simulink model "UIO_example_EEG"  (R2019b)
settings: Solver=FixedStepAuto  StartTime=0.0  StopTime=3  FixedStep=dt  RelTol=1e-3
values from neighbouring files (symbols this model uses):
  B2 = [68245 0 0;0 -2 0;0 0 2;0 232.75 0; 0 0 -232.75]    [UIO_adaptive_example.m]    (also in UIO_adaptive_example_2.m = [1;0;1;0]; UIO_adaptive_example_EEG.m = ones(opt_order,1); UIO_adaptive_example_EEG_Balas_2ch.m = ones(opt_order,1); UIO_adaptive_example_EEG_ch2.m = ones(opt_order,1))
  F = B2'*P/(C)    [UIO_adaptive_example_2.m]    (also in UIO_adaptive_example_EEG.m = B2'*P/(C_data{opt_order}); UIO_adaptive_example_EEG_ch2.m = B2'*P/(C_data{opt_order}); UIO_adaptive_example_EEG_ch2_DEAP.m = B2'*P/(C_data{opt_order}); UIO_adaptive_example_EEG_ch2_ECEO.m = B2'*P/(C_data{opt_order}))
  Gamma = 20    [UIO_adaptive_example_2.m]    (also in UIO_adaptive_example_EEG.m = 0.001; UIO_adaptive_example_EEG_ch2.m = loop(i); UIO_adaptive_example_EEG_ch2_DEAP.m = loop(i); UIO_adaptive_example_EEG_ch2_ECEO.m = loop(i))
  L = inv(P)*Y    [UIO_adaptive_example.m]    (also in UIO_adaptive_example_2.m; UIO_adaptive_example_EEG.m; UIO_adaptive_example_EEG_ch2.m; UIO_adaptive_example_EEG_ch2_DEAP.m)
  opt_order = 20    [UIO_adaptive_example_EEG.m]    (also in UIO_adaptive_example_EEG_Balas_2ch.m = 4; UIO_adaptive_example_EEG_ch2.m = 4; UIO_adaptive_example_EEG_ch2_DEAP.m = 4; UIO_adaptive_example_EEG_ch2_ECEO.m = 4)
settings Model: Creator=Tris  LastModifiedBy=Tris
settings DataIOCC: ExternalInput=Y_sim1, Y_sim2, Y_sim3, Y_sim4, Y_sim5, Y_sim6  LoadExternalInput=on

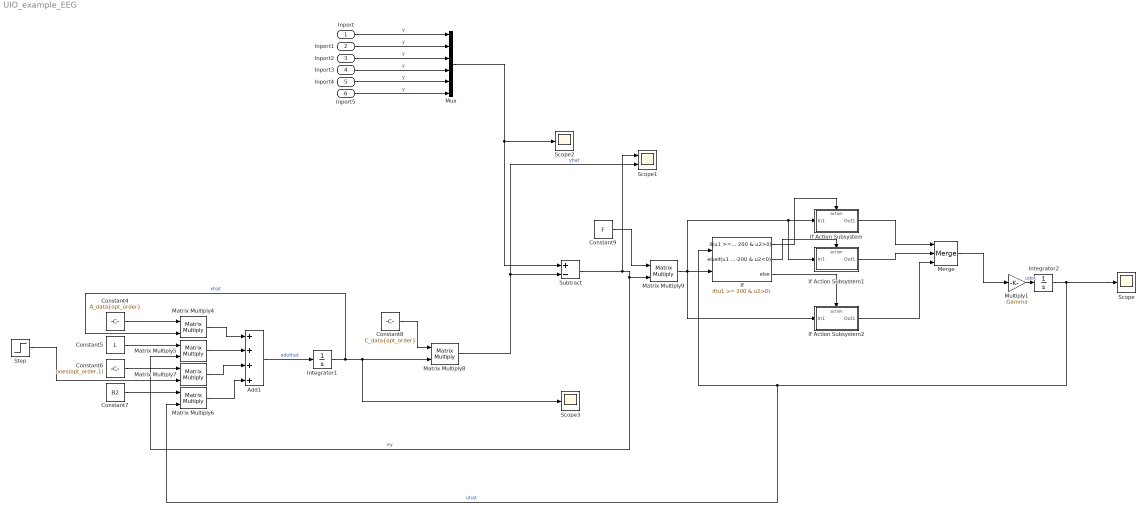
== system UIO_example_EEG ==
  Inport : Inport
  Inport1 : Inport  Port=2
  Inport2 : Inport  Port=3
  Inport3 : Inport  Port=4
  Inport4 : Inport  Port=5
  Inport5 : Inport  Port=6
  Add1 : Sum  Inputs=++++
  Constant4 : Constant  Value=A_data{opt_order}  VectorParams1D=off
  Constant5 : Constant  Value=L  VectorParams1D=off
  Constant6 : Constant  Value=ones(opt_order,1)  VectorParams1D=off
  Constant7 : Constant  Value=B2  VectorParams1D=off
  Constant8 : Constant  Value=C_data{opt_order}  VectorParams1D=off
  Constant9 : Constant  Value=F  VectorParams1D=off
  If : If  NumInputs=2  IfExpression=u1 >= 200 & u2>0  ElseIfExpressions=u1 <= -200 & u2<0
  If Action Subsystem : Subsystem  TreatAsAtomicUnit=on
  If Action Subsystem1 : Subsystem  TreatAsAtomicUnit=on
  If Action Subsystem2 : Subsystem  TreatAsAtomicUnit=on
  Integrator1 : Integrator
  Integrator2 : Integrator  InitialCondition=2
  Matrix Multiply{4..9} (6 alike) : Product  Multiplication=Matrix(*)
  Merge : Merge  Inputs=3
  Multiply1 : Gain  Gain=Gamma
  Mux : Mux  Inputs=6
  Scope : Scope
  Scope1 : Scope  NumInputPorts=2
  Scope2 : Scope
  Scope3 : Scope
  Step : Step  After=0  SampleTime=0
  Subtract : Sum  Inputs=+-
  wires:
  Matrix Multiply5/1 -> Add1/2
  Matrix Multiply4/1 -> Add1/1
  Matrix Multiply7/1 -> Add1/3
  Matrix Multiply6/1 -> Add1/4
  Constant4/1 -> Matrix Multiply4/1
  Constant5/1 -> Matrix Multiply5/1
  Constant6/1 -> Matrix Multiply7/1
  Constant7/1 -> Matrix Multiply6/1
  Add1/1 -> Integrator1/1  "xdothat"
  Integrator1/1 -> Scope3/1, Matrix Multiply8/2, Matrix Multiply4/2  "xhat"
  Matrix Multiply8/1 -> Scope1/2, Subtract/2  "yhat"
  Subtract/1 -> Scope1/1, Matrix Multiply5/2, Matrix Multiply9/2  "ey"
  Matrix Multiply9/1 -> If/2, If Action Subsystem2/1(In1), If Action Subsystem1/1(In1), If Action Subsystem/1(In1)
  Integrator2/1 -> Scope/1, Matrix Multiply6/2, If/1  "uhat"
  Step/1 -> Matrix Multiply7/2
  Constant8/1 -> Matrix Multiply8/1
  Constant9/1 -> Matrix Multiply9/1
  Multiply1/1 -> Integrator2/1  "udot"
  If/1 -> If Action Subsystem/Action
  If/2 -> If Action Subsystem1/Action
  If/3 -> If Action Subsystem2/Action
  If Action Subsystem1/1(Out1) -> Merge/2
  If Action Subsystem2/1(Out1) -> Merge/3
  Merge/1 -> Multiply1/1
  If Action Subsystem/1(Out1) -> Merge/1
  Inport/1 -> Mux/1  "y"
  Inport1/1 -> Mux/2  "y"
  Inport2/1 -> Mux/3  "y"
  Inport3/1 -> Mux/4  "y"
  Inport4/1 -> Mux/5  "y"
  Inport5/1 -> Mux/6  "y"
  Mux/1 -> Subtract/1, Scope2/1

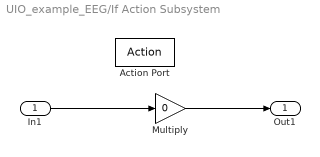
== system UIO_example_EEG/If Action Subsystem ==
  In1 : Inport
  Action Port : ActionPort  ActionPortLabel=if(u1 >= 200 & u2>0)
  Multiply : Gain  Gain=0
  Out1 : Outport
  wires:
  In1/1 -> Multiply/1
  Multiply/1 -> Out1/1

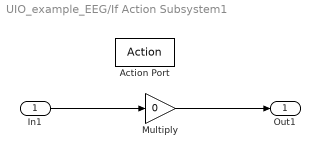
== system UIO_example_EEG/If Action Subsystem1 ==
  In1 : Inport
  Action Port : ActionPort  ActionPortLabel=elseif(u1 <= -200 & u2<0)
  Multiply : Gain  Gain=0
  Out1 : Outport
  wires:
  In1/1 -> Multiply/1
  Multiply/1 -> Out1/1

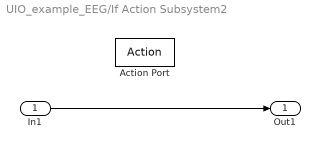
== system UIO_example_EEG/If Action Subsystem2 ==
  In1 : Inport
  Action Port : ActionPort  ActionPortLabel=else
  Out1 : Outport
  wires:
  In1/1 -> Out1/1
